simulink model "simul_new1"  (R2017b)
settings: Solver=VariableStepAuto  StartTime=0.0  StopTime=50  RelTol=1e-3
values from neighbouring files (symbols this model uses):
  F1 = ft(1)    [Untitled_new.m]
  F2 = ft(2)    [Untitled_new.m]
  F3 = ft(3)    [Untitled_new.m]
  F4 = ft(4)    [Untitled_new.m]
  K = Tau/m    (= 0.0252105077396)    [Untitled_new.m]
  Kdm = Kpm*Tdm    [Untitled_new.m]
  Kim = Kpm/Tim    [Untitled_new.m]
  Kpm = Kc*Md*cos(fid)    [Untitled_new.m]
  T = Ts    (= 0.01)    [Untitled_new.m]
  Tau = (m/(rho*A*Cd*(u0+uw)))    (= 126.052538698)    [Untitled_new.m]
libraries: cstblocks x1, simulink x1
settings Model: Creator=Student  LastModifiedBy=Student

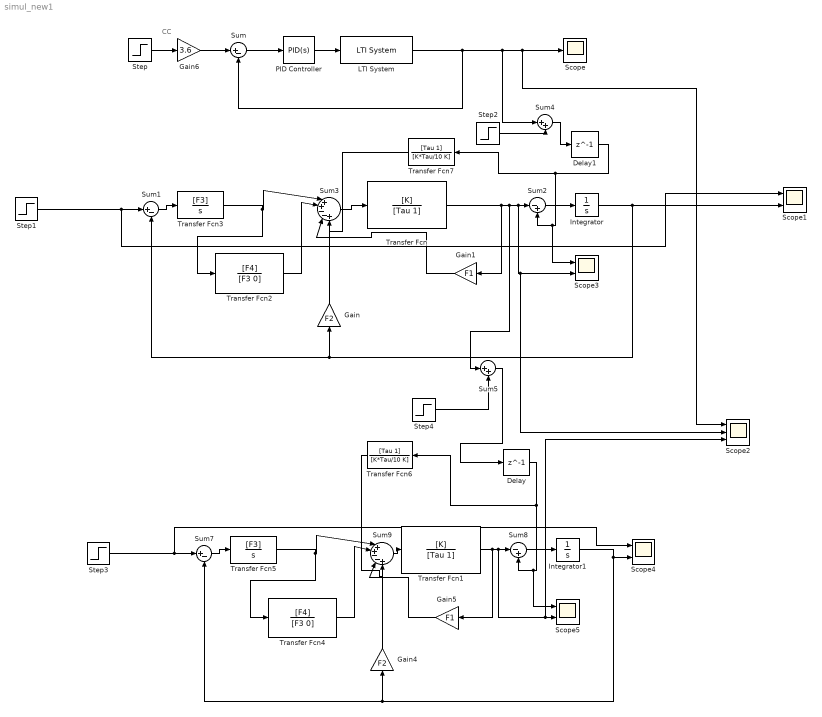
== system simul_new1 ==
  note: CC
  Delay : Delay  DelayLength=1  SampleTime=T
  Delay1 : Delay  DelayLength=1  InitialCondition=0  SampleTime=T
  Gain : Gain  Gain=F2
  Gain1 : Gain  Gain=F1
  Gain4 : Gain  Gain=F2
  Gain5 : Gain  Gain=F1
  Gain6 : Gain  Gain=3.6
  Integrator : Integrator
  Integrator1 : Integrator
  LTI System : cstblocks/LTI System  sys=Gm  IC=[]
  PID Controller : simulink/Continuous/PID Controller  Controller=PID  TimeDomain=Continuous-time  SampleTime=-1  IntegratorMethod=Forward Euler  FilterMethod=Forward Euler  Form=Parallel  UseFilter=on  ControllerParametersSource=internal  P=Kpm  I=Kim  D=Kdm  N=1.5  InitialConditionSource=internal  InitialConditionForIntegrator=0  InitialConditionForFilter=0  ExternalReset=none  LimitOutput=off  UpperSaturationLimit=inf  LowerSaturationLimit=-inf  LinearizeAsGain=on  AntiWindupMode=none  Kb=1  TrackingMode=off  Kt=1  PParamMin=[]  PParamMax=[]  IParamMin=[]  IParamMax=[]  DParamMin=[]  DParamMax=[]  NParamMin=[]  NParamMax=[]  KbParamMin=[]  KbParamMax=[]  KtParamMin=[]  KtParamMax=[]  POutMin=[]  POutMax=[]  IOutMin=[]  IOutMax=[]  DOutMin=[]  DOutMax=[]  NOutMin=[]  NOutMax=[]  KbOutMin=[]  KbOutMax=[]  KtOutMin=[]  KtOutMax=[]  IntegratorOutMin=[]  IntegratorOutMax=[]  FilterOutMin=[]  FilterOutMax=[]  SumOutMin=[]  SumOutMax=[]  SumI1OutMin=[]  SumI1OutMax=[]  SumI2OutMin=[]  SumI2OutMax=[]  SumI3OutMin=[]  SumI3OutMax=[]  SumDOutMin=[]  SumDOutMax=[]  SaturationOutMin=[]  SaturationOutMax=[]  IntegratorContinuousStateAttributes=''  IntegratorStateMustResolveToSignalObject=off  IntegratorRTWStateStorageClass=Auto  FilterContinuousStateAttributes=''  FilterStateMustResolveToSignalObject=off  FilterRTWStateStorageClass=Auto  DifferentiatorICPrevScaledInput=0  DifferentiatorOutMin=[]  DifferentiatorOutMax=[]  InitialConditionSetting=State (most efficient)  FilterDiffOutCoefMin=[]  FilterDiffOutCoefMax=[]  SumDenOutMin=[]  SumDenOutMax=[]  SumNumOutMin=[]  SumNumOutMax=[]  ReciprocalOutMin=[]  ReciprocalOutMax=[]  DivideOutMin=[]  DivideOutMax=[]  TunerSelectOption=Transfer Function Based (PID Tuner App)
  Scope : Scope
  Scope{1,3..5} (4 alike) : Scope  NumInputPorts=2
  Scope2 : Scope  NumInputPorts=3
  Step : Step  Time=0  After=20  SampleTime=0.01
  Step1 : Step  Time=0  Before=10  After=20  SampleTime=T
  Step2 : Step  Time=5  Before=5  After=0  SampleTime=0
  Step3 : Step  Time=0  Before=20  After=30  SampleTime=T
  Step4 : Step  Time=5  Before=5  After=0  SampleTime=0
  Sum : Sum  Inputs=|+-
  Sum1 : Sum  Inputs=|+-
  Sum2 : Sum  Inputs=|-+
  Sum3 : Sum  Inputs=|++--+
  Sum4 : Sum  Inputs=|++
  Sum5 : Sum  Inputs=|++
  Sum7 : Sum  Inputs=|+-
  Sum8 : Sum  Inputs=|-+
  Sum9 : Sum  Inputs=|++--+
  Transfer Fcn : TransferFcn  Numerator=[K]  Denominator=[Tau 1]
  Transfer Fcn1 : TransferFcn  Numerator=[K]  Denominator=[Tau 1]
  Transfer Fcn2 : TransferFcn  Numerator=[F4]  Denominator=[F3 0]
  Transfer Fcn3 : TransferFcn  Numerator=[F3]  Denominator=[1 0]
  Transfer Fcn4 : TransferFcn  Numerator=[F4]  Denominator=[F3 0]
  Transfer Fcn5 : TransferFcn  Numerator=[F3]  Denominator=[1 0]
  Transfer Fcn6 : TransferFcn  Numerator=[Tau 1]  Denominator=[K*Tau/10 K]
  Transfer Fcn7 : TransferFcn  Numerator=[Tau 1]  Denominator=[K*Tau/10 K]
  wires:
  Step/1 -> Gain6/1
  Sum/1 -> PID Controller/1
  PID Controller/1 -> LTI System/1
  Sum2/1 -> Integrator/1
  Delay1/1 -> Transfer Fcn7/1, Scope3/1, Sum2/2
  Sum3/1 -> Transfer Fcn/1
  Gain/1 -> Sum3/3
  Integrator/1 -> Gain/1, Sum1/2, Scope1/2
  Gain1/1 -> Sum3/4
  Step1/1 -> Scope1/1, Sum1/1
  Sum1/1 -> Transfer Fcn3/1
  Transfer Fcn3/1 -> Transfer Fcn2/1, Sum3/1
  Transfer Fcn2/1 -> Sum3/2
  Transfer Fcn4/1 -> Sum9/2
  Transfer Fcn5/1 -> Transfer Fcn4/1, Sum9/1
  Sum7/1 -> Transfer Fcn5/1
  Gain5/1 -> Sum9/4
  Sum9/1 -> Transfer Fcn1/1
  Delay/1 -> Transfer Fcn6/1, Scope5/1, Sum8/2
  Step3/1 -> Scope4/1, Sum7/1
  Sum8/1 -> Integrator1/1
  Integrator1/1 -> Scope4/2, Gain4/1, Sum7/2
  Transfer Fcn1/1 -> Sum8/1, Scope2/3, Scope5/2, Gain5/1
  Gain4/1 -> Sum9/3
  Transfer Fcn7/1 -> Sum3/5
  Transfer Fcn6/1 -> Sum9/5
  Gain6/1 -> Sum/1
  LTI System/1 -> Sum/2, Sum4/1, Scope2/1, Scope/1
  Transfer Fcn/1 -> Gain1/1, Sum5/1, Scope2/2, Scope3/2, Sum2/1
  Sum5/1 -> Delay/1
  Step4/1 -> Sum5/2
  Sum4/1 -> Delay1/1
  Step2/1 -> Sum4/2
